simulink model "sito_three_output_buck_full"  (R2025a)
settings: Solver=ode23tb  StartTime=0  StopTime=0.01  MaxStep=1e-6  RelTol=1e-3
libraries: spsGroundLib x11, spsSeriesRLCBranchLib x7, spsDiodeLib x4, spsIdealSwitchLib x3, spsVoltageMeasurementLib x3, spsCurrentMeasurementLib x1, simulink x1, spsDCVoltageSourceLib x1, sps_lib x1
settings Model: Creator=GrowU  LastModifiedBy=GrowU

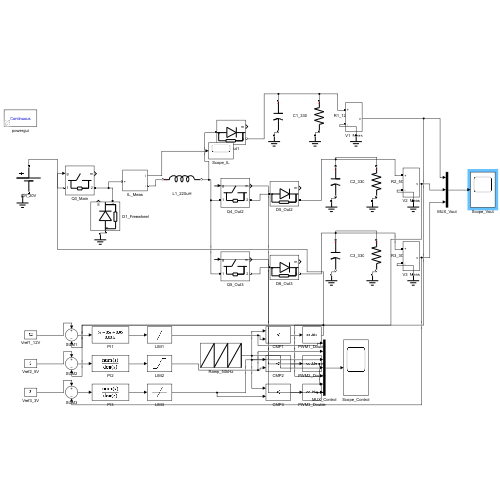
[thumbnail: Simulink's stored preview of the top-level diagram]
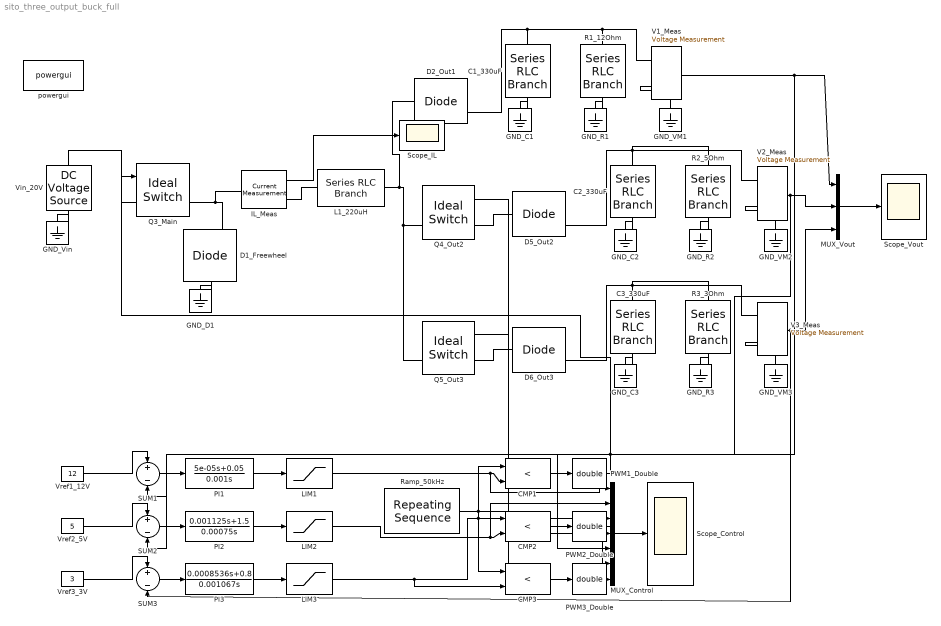
== system sito_three_output_buck_full ==
  C1_330uF : spsSeriesRLCBranchLib/Series RLC Branch  LConnTagsString=__new0  RConnTagsString=__new0  BranchType=C  Resistance=1  Inductance=1e-3  SetiL0=off  InitialCurrent=0  Capacitance=0.00033  Setx0=off  InitialVoltage=0  Measurements=None
  C2_330uF : spsSeriesRLCBranchLib/Series RLC Branch  LConnTagsString=__new0  RConnTagsString=__new0  BranchType=C  Resistance=1  Inductance=1e-3  SetiL0=off  InitialCurrent=0  Capacitance=0.00033  Setx0=off  InitialVoltage=0  Measurements=None
  C3_330uF : spsSeriesRLCBranchLib/Series RLC Branch  LConnTagsString=__new0  RConnTagsString=__new0  BranchType=C  Resistance=1  Inductance=1e-3  SetiL0=off  InitialCurrent=0  Capacitance=0.00033  Setx0=off  InitialVoltage=0  Measurements=None
  CMP1 : RelationalOperator  Operator=<  OutDataTypeStr=boolean  RndMeth=Simplest  InputSameDT=off
  CMP2 : RelationalOperator  Operator=<  OutDataTypeStr=boolean  RndMeth=Simplest  InputSameDT=off
  CMP3 : RelationalOperator  Operator=<  OutDataTypeStr=boolean  RndMeth=Simplest  InputSameDT=off
  D1_Freewheel : spsDiodeLib/Diode  Ron=0.001  Lon=0  Vf=0  IC=0  UseSnubber=off  Rs=1000000  Cs=inf  Measurements=on
  D2_Out1 : spsDiodeLib/Diode  Ron=0.001  Lon=0  Vf=0  IC=0  UseSnubber=off  Rs=1000000  Cs=inf  Measurements=on
  D5_Out2 : spsDiodeLib/Diode  Ron=0.001  Lon=0  Vf=0  IC=0  UseSnubber=off  Rs=1000000  Cs=inf  Measurements=on
  D6_Out3 : spsDiodeLib/Diode  Ron=0.001  Lon=0  Vf=0  IC=0  UseSnubber=off  Rs=1000000  Cs=inf  Measurements=on
  GND_C1 : spsGroundLib/Ground  LConnTagsString=a
  GND_C2 : spsGroundLib/Ground  LConnTagsString=a
  GND_C3 : spsGroundLib/Ground  LConnTagsString=a
  GND_D1 : spsGroundLib/Ground  LConnTagsString=a
  GND_R1 : spsGroundLib/Ground  LConnTagsString=a
  GND_R2 : spsGroundLib/Ground  LConnTagsString=a
  GND_R3 : spsGroundLib/Ground  LConnTagsString=a
  GND_VM1 : spsGroundLib/Ground  LConnTagsString=a
  GND_VM2 : spsGroundLib/Ground  LConnTagsString=a
  GND_VM3 : spsGroundLib/Ground  LConnTagsString=a
  GND_Vin : spsGroundLib/Ground  LConnTagsString=a
  IL_Meas : spsCurrentMeasurementLib/Current Measurement  PhasorSimulation=off  OutputType=Complex  PSBequivalent=0
  L1_220uH : spsSeriesRLCBranchLib/Series RLC Branch  LConnTagsString=__new0  RConnTagsString=__new0  BranchType=L  Resistance=0  Inductance=0.00022  SetiL0=off  InitialCurrent=0  Capacitance=1e-6  Setx0=off  InitialVoltage=0  Measurements=Branch current
  LIM1 : Saturate  UpperLimit=1  LowerLimit=0
  LIM2 : Saturate  UpperLimit=1  LowerLimit=0
  LIM3 : Saturate  UpperLimit=1  LowerLimit=0
  MUX_Control : Mux  Inputs=7
  MUX_Vout : Mux  Inputs=3
  PI1 : TransferFcn  Numerator=[5e-05 0.05]  Denominator=[0.001 0]
  PI2 : TransferFcn  Numerator=[0.001125 1.5]  Denominator=[0.00075 0]
  PI3 : TransferFcn  Numerator=[0.0008536 0.8]  Denominator=[0.001067 0]
  PWM1_Double : DataTypeConversion  OutDataTypeStr=double  SaturateOnIntegerOverflow=off  RndMeth=Floor
  PWM2_Double : DataTypeConversion  OutDataTypeStr=double  SaturateOnIntegerOverflow=off  RndMeth=Floor
  PWM3_Double : DataTypeConversion  OutDataTypeStr=double  SaturateOnIntegerOverflow=off  RndMeth=Floor
  Q3_Main : spsIdealSwitchLib/Ideal Switch  Ron=0.0048  Lon=0  IC=0  Rs=1000000  Cs=inf  Measurements=on
  Q4_Out2 : spsIdealSwitchLib/Ideal Switch  Ron=0.0048  Lon=0  IC=0  Rs=1000000  Cs=inf  Measurements=on
  Q5_Out3 : spsIdealSwitchLib/Ideal Switch  Ron=0.0048  Lon=0  IC=0  Rs=1000000  Cs=inf  Measurements=on
  R1_12Ohm : spsSeriesRLCBranchLib/Series RLC Branch  LConnTagsString=__new0  RConnTagsString=__new0  BranchType=R  Resistance=12  Inductance=1e-3  SetiL0=off  InitialCurrent=0  Capacitance=1e-6  Setx0=off  InitialVoltage=0  Measurements=None
  R2_5Ohm : spsSeriesRLCBranchLib/Series RLC Branch  LConnTagsString=__new0  RConnTagsString=__new0  BranchType=R  Resistance=5  Inductance=1e-3  SetiL0=off  InitialCurrent=0  Capacitance=1e-6  Setx0=off  InitialVoltage=0  Measurements=None
  R3_3Ohm : spsSeriesRLCBranchLib/Series RLC Branch  LConnTagsString=__new0  RConnTagsString=__new0  BranchType=R  Resistance=3  Inductance=1e-3  SetiL0=off  InitialCurrent=0  Capacitance=1e-6  Setx0=off  InitialVoltage=0  Measurements=None
  Ramp_50kHz : simulink/Sources/Repeating Sequence  rep_seq_t=[0 2e-05]  rep_seq_y=[0 1]
  SUM1 : Sum  Inputs=+-
  SUM2 : Sum  Inputs=+-
  SUM3 : Sum  Inputs=+-
  Scope_Control : Scope
  Scope_IL : Scope
  Scope_Vout : Scope
      settings: ActiveDisplayYMinimum=-3.5569303305364421  ActiveDisplayYMaximum=24.322460549960507
  V1_Meas : spsVoltageMeasurementLib/Voltage Measurement  PhasorSimulation=off  OutputType=Complex  PSBequivalent=0
  V2_Meas : spsVoltageMeasurementLib/Voltage Measurement  PhasorSimulation=off  OutputType=Complex  PSBequivalent=0
  V3_Meas : spsVoltageMeasurementLib/Voltage Measurement  PhasorSimulation=off  OutputType=Complex  PSBequivalent=0
  Vin_20V : spsDCVoltageSourceLib/DC Voltage Source  Amplitude=20  Measurements=None
  Vref1_12V : Constant  Value=12
  Vref2_5V : Constant  Value=5
  Vref3_3V : Constant  Value=3
  powergui : sps_lib/powergui  Priority=1  SimulationMode=Continuous  SampleTime=50e-6  frequency=60  Iterations=50  frequencyindice=0  Pbase=100e6  ErrMax=1e-4  UnitsV=kV  UnitsW=MW  buscounter=0  FunctionMessages=off  echomessages=off  EnableUseOfTLC=off  CurrentSourceSwitches=off  DisableSnubberDevices=off  DisableRonSwitches=off  DisableVfSwitches=off  DisplayEquations=off  AutomaticDiscreteSolvers=off  SolverType=Tustin/Backward Euler (TBE)  Interpol=off  ExternalGateDelay=off  methode=off  Ts=100  x0status=blocks  SPID=on  SwTol=0  HookPort=off  NonlinearTolerance=1e-4  nMaxIteration=100  ContinueOnMaxIteration=off  RestoreLinks=warning  ResistiveCurrentMeasurement=off  Frange=[0:2:500]  Ylog=off  Xlog=on  ShowGrid=off  save=off  variable=ZData  structure=0  ZoomFFT=off  StartTime=0.0  cycles=1  DisplayStyle=1  fundamental=60  FreqAxis=off  MaxFrequency=1000  frequencyindicesteady=1  RmsSteady=1  display=off
  wires:
  Vref1_12V/1 -> SUM1/1
  V1_Meas/1 -> SUM1/2, MUX_Vout/1
  SUM1/1 -> PI1/1
  PI1/1 -> LIM1/1
  Vref2_5V/1 -> SUM2/1
  V2_Meas/1 -> SUM2/2, MUX_Vout/2
  SUM2/1 -> PI2/1
  PI2/1 -> LIM2/1
  Vref3_3V/1 -> SUM3/1
  V3_Meas/1 -> SUM3/2, MUX_Vout/3
  SUM3/1 -> PI3/1
  PI3/1 -> LIM3/1
  Ramp_50kHz/1 -> CMP2/1, CMP3/1, CMP1/1, MUX_Control/4
  LIM1/1 -> CMP1/2, MUX_Control/1
  LIM2/1 -> CMP2/2, MUX_Control/2
  LIM3/1 -> CMP3/2, MUX_Control/3
  CMP1/1 -> PWM1_Double/1
  CMP2/1 -> PWM2_Double/1
  CMP3/1 -> PWM3_Double/1
  PWM1_Double/1 -> Q3_Main/1, MUX_Control/5
  PWM2_Double/1 -> Q4_Out2/1, MUX_Control/6
  PWM3_Double/1 -> Q5_Out3/1, MUX_Control/7
  MUX_Vout/1 -> Scope_Vout/1
  MUX_Control/1 -> Scope_Control/1
  IL_Meas/1 -> Scope_IL/1
  connections:
  Vin_20V/RConn1 -- Q3_Main/LConn1
  Vin_20V/LConn1 -- GND_Vin/LConn1
  IL_Meas/LConn1 -- Q3_Main/RConn1 -- D1_Freewheel/RConn1
  IL_Meas/RConn1 -- L1_220uH/LConn1
  D1_Freewheel/LConn1 -- GND_D1/LConn1
  D2_Out1/LConn1 -- L1_220uH/RConn1 -- Q4_Out2/LConn1 -- Q5_Out3/LConn1
  D2_Out1/RConn1 -- V1_Meas/LConn1 -- R1_12Ohm/LConn1 -- C1_330uF/LConn1
  C1_330uF/RConn1 -- GND_C1/LConn1
  R1_12Ohm/RConn1 -- GND_R1/LConn1
  V1_Meas/LConn2 -- GND_VM1/LConn1
  Q4_Out2/RConn1 -- D5_Out2/LConn1
  D5_Out2/RConn1 -- C2_330uF/LConn1 -- V2_Meas/LConn1 -- R2_5Ohm/LConn1
  C2_330uF/RConn1 -- GND_C2/LConn1
  R2_5Ohm/RConn1 -- GND_R2/LConn1
  V2_Meas/LConn2 -- GND_VM2/LConn1
  Q5_Out3/RConn1 -- D6_Out3/LConn1
  D6_Out3/RConn1 -- C3_330uF/LConn1 -- V3_Meas/LConn1 -- R3_3Ohm/LConn1
  C3_330uF/RConn1 -- GND_C3/LConn1
  R3_3Ohm/RConn1 -- GND_R3/LConn1
  V3_Meas/LConn2 -- GND_VM3/LConn1
